simulink model "PP_s_inv_L"  (R2023b)
settings: Solver=VariableStepAuto  StartTime=0.0  StopTime=10.0  RelTol=1e-3
values from neighbouring files (symbols this model uses):
  A = [0 1; 9.81 -0.1]    [WP2.m]
  B = [0; 1]    [WP2.m]
  K = [k1 k2 ki]    [WP2.m]
  kr = -1/(C*inv(A-B*K)*B)    [WP2.m]
  rl = 0    [WP2.m]
settings Model: Creator=giova  LastModifiedBy=Principale

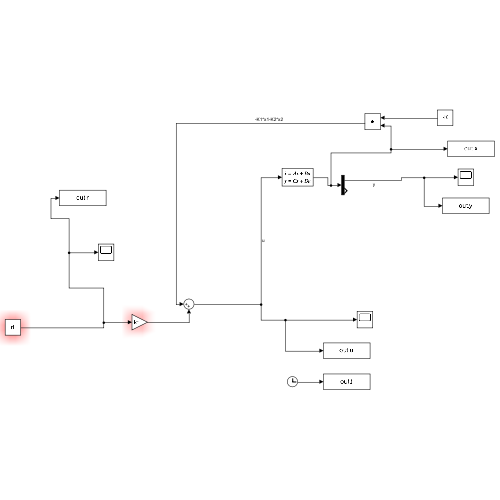
[thumbnail: Simulink's stored preview of the top-level diagram]
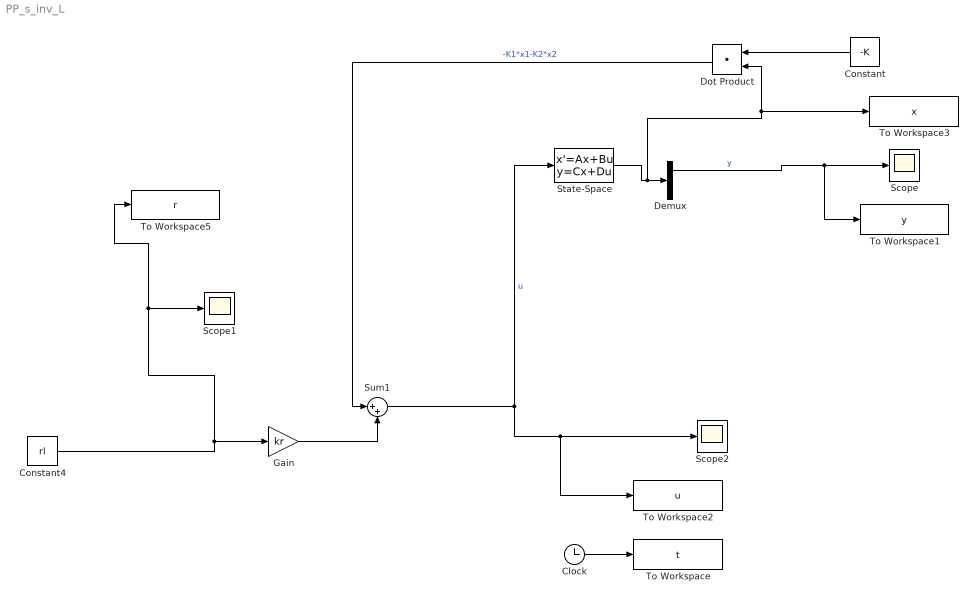
== system PP_s_inv_L ==
  Clock : Clock
  Constant : Constant  Value=-K
  Constant4 : Constant  Value=rl
  Demux : Demux  Outputs=2
  Dot Product : DotProduct  OutDataTypeStr=Inherit: Inherit via internal rule
  Gain : Gain  Gain=kr
  Scope : Scope
  Scope1 : Scope
  Scope2 : Scope
  State-Space : StateSpace  A=A  B=B  C=eye(2)  D=[0;0]  InitialCondition=[pi, 0]
  Sum1 : Sum  Inputs=|++
  To Workspace : ToWorkspace  VariableName=t  SampleTime=-1
  To Workspace1 : ToWorkspace  VariableName=y  SampleTime=-1
  To Workspace2 : ToWorkspace  VariableName=u  SampleTime=-1
  To Workspace3 : ToWorkspace  VariableName=x  SampleTime=-1
  To Workspace5 : ToWorkspace  VariableName=r  SampleTime=-1
  wires:
  Sum1/1 -> Scope2/1, To Workspace2/1, State-Space/1  "u"
  Constant4/1 -> Scope1/1, To Workspace5/1, Gain/1
  Gain/1 -> Sum1/2
  Clock/1 -> To Workspace/1
  Constant/1 -> Dot Product/1
  State-Space/1 -> To Workspace3/1, Dot Product/2, Demux/1
  Demux/1 -> To Workspace1/1, Scope/1  "y"
  Dot Product/1 -> Sum1/1  "-K1*x1-K2*x2"
